simulink model "a"  (R2022b)
settings: Solver=VariableStepAuto  StartTime=0.0  StopTime=10.0  RelTol=1e-3
values from neighbouring files (symbols this model uses):
  B = .1    (= 0.1)    [Lab06.m]    (also in s270874.mat)
  g = 9.81    [Lab06.m]    (also in s270874.mat)
  l = .5    (= 0.5)    [Lab06.m]    (also in s270874.mat)
  m = .1    (= 0.1)    [Lab06.m]    (also in s270874.mat)
  theta0 = pi/2 - 1e-2    (= 1.56079632679)    [Lab06.m]    (also in s270874.mat)
  u_bar = l*m*g    (= 0.4905)    [Lab06.m]    (also in s270874.mat)
  velocity0 = 0    [Lab06.m]    (also in s270874.mat)
settings Model: Creator=franc  LastModifiedBy=franc

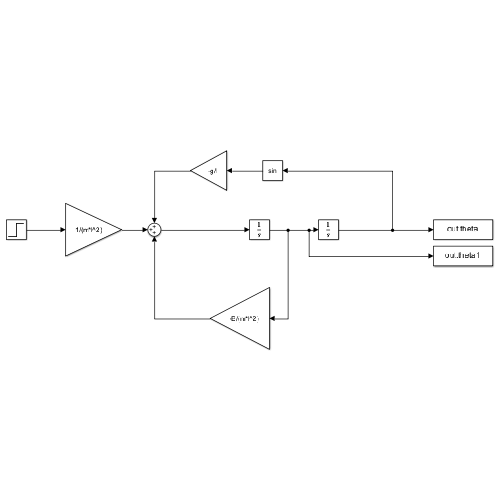
[thumbnail: Simulink's stored preview of the top-level diagram]
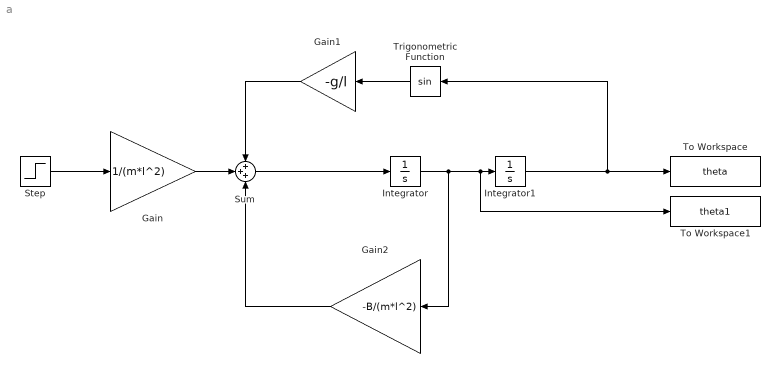
== system a ==
  Gain : Gain  Gain=1/(m*l^2)
  Gain1 : Gain  Gain=-g/l
  Gain2 : Gain  Gain=-B/(m*l^2)
  Integrator : Integrator  InitialCondition=velocity0
  Integrator1 : Integrator  InitialCondition=theta0
  Step : Step  Time=0  After=u_bar  SampleTime=0
  Sum : Sum  Inputs=+++
  To Workspace : ToWorkspace  VariableName=theta  SaveFormat=Timeseries  SampleTime=-1
  To Workspace1 : ToWorkspace  VariableName=theta1  SaveFormat=Timeseries  SampleTime=-1
  Trigonometric Function : Trigonometry
  wires:
  Step/1 -> Gain/1
  Sum/1 -> Integrator/1
  Trigonometric Function/1 -> Gain1/1
  Integrator/1 -> Gain2/1, To Workspace1/1, Integrator1/1
  Integrator1/1 -> Trigonometric Function/1, To Workspace/1
  Gain/1 -> Sum/2
  Gain1/1 -> Sum/1
  Gain2/1 -> Sum/3
